simulink model "simsevenlevelmulti"  (R2023a)
settings: Solver=VariableStepAuto  StartTime=0.0  StopTime=10.0  RelTol=1e-3
libraries: spsIGBTDiodeLib x12, simulink x6, spsDCVoltageSourceLib x3, spsSeriesRLCBranchLib x1, spsVoltageMeasurementLib x1, spspowerguiLib x1
settings Model: Creator=banof  LastModifiedBy=banof

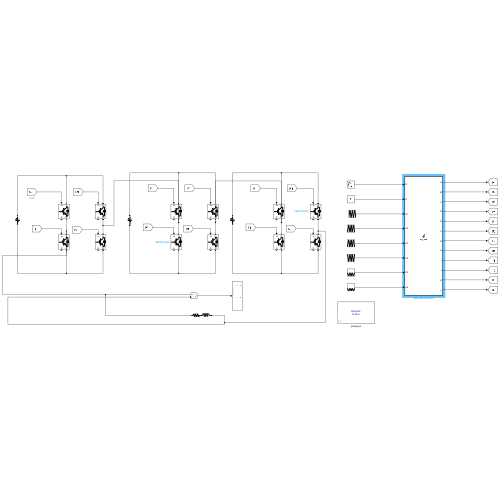
[thumbnail: Simulink's stored preview of the top-level diagram]
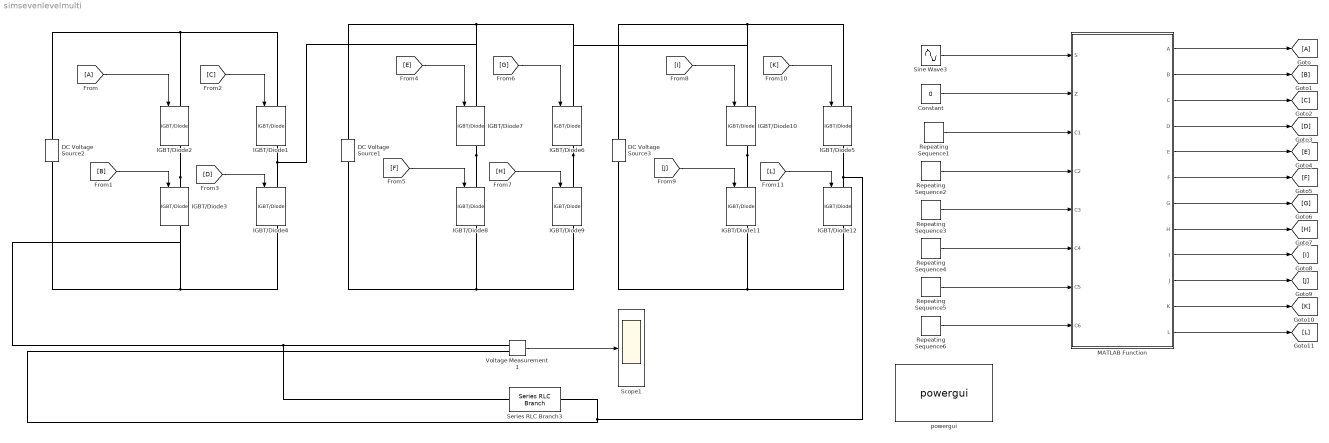
== system simsevenlevelmulti ==
  Constant : Constant  Value=0
  DC Voltage Source1 : spsDCVoltageSourceLib/DC Voltage Source  Amplitude=100  Measurements=None
  DC Voltage Source2 : spsDCVoltageSourceLib/DC Voltage Source  Amplitude=100  Measurements=None
  DC Voltage Source3 : spsDCVoltageSourceLib/DC Voltage Source  Amplitude=100  Measurements=None
  From : From
  Goto : Goto
  IGBT/Diode{1..12} (12 alike) : spsIGBTDiodeLib/IGBT//Diode  Ron=1e-3  Rs=1e5  Cs=inf  Measurements=on
  MATLAB Function : MATLAB Function  TreatAsAtomicUnit=on
  Repeating Sequence1 : simulink/Sources/Repeating Sequence  rep_seq_t=[0 0.5/1000 1/1000]  rep_seq_y=[0 0.3334 0]
  Repeating Sequence2 : simulink/Sources/Repeating Sequence  rep_seq_t=[0 0.5/1000 1/1000]  rep_seq_y=[0.3334 0.6667 0.3334]
  Repeating Sequence3 : simulink/Sources/Repeating Sequence  rep_seq_t=[0 0.5/1000 1/1000]  rep_seq_y=[0.6667 1.0000 0.6667]
  Repeating Sequence4 : simulink/Sources/Repeating Sequence  rep_seq_t=[0 0.5/1000 1/1000]  rep_seq_y=[0 -0.3334 0]
  Repeating Sequence5 : simulink/Sources/Repeating Sequence  rep_seq_t=[0 0.5/1000 1/1000]  rep_seq_y=[-0.3334 -0.6667 -0.3334]
  Repeating Sequence6 : simulink/Sources/Repeating Sequence  rep_seq_t=[0 0.5/1000 1/1000]  rep_seq_y=[-0.6667 -1 -0.6667]
  Scope1 : Scope
  Series RLC Branch3 : spsSeriesRLCBranchLib/Series RLC Branch  LConnTagsString=__new0  RConnTagsString=__new0  BranchType=RL  Resistance=100  Inductance=100e-3  SetiL0=off  InitialCurrent=0  Capacitance=1e-6  Setx0=off  InitialVoltage=0  Measurements=None
  Sine Wave3 : Sin  Frequency=2*pi*50
  Voltage Measurement1 : spsVoltageMeasurementLib/Voltage Measurement  PhasorSimulation=off  OutputType=Complex  PSBequivalent=0
  powergui : spspowerguiLib/powergui  Priority=1  SimulationMode=Discrete  SampleTime=1e-6  frequency=60  Iterations=50  frequencyindice=0  Pbase=100e6  ErrMax=1e-4  UnitsV=kV  UnitsW=MW  buscounter=0  FunctionMessages=off  echomessages=off  EnableUseOfTLC=off  CurrentSourceSwitches=off  DisableSnubberDevices=off  DisableRonSwitches=off  DisableVfSwitches=off  DisplayEquations=off  AutomaticDiscreteSolvers=off  SolverType=Tustin/Backward Euler (TBE)  Interpol=off  ExternalGateDelay=off  methode=off  Ts=100  x0status=blocks  SPID=on  SwTol=0  HookPort=off  NonlinearTolerance=1e-4  nMaxIteration=100  ContinueOnMaxIteration=off  RestoreLinks=warning  ResistiveCurrentMeasurement=off  Frange=[0:2:500]  Ylog=off  Xlog=on  ShowGrid=off  save=off  variable=ZData  structure=0  ZoomFFT=off  StartTime=0.0  cycles=1  DisplayStyle=1  fundamental=60  FreqAxis=off  MaxFrequency=1000  frequencyindicesteady=1  RmsSteady=1  display=off
  wires:
  MATLAB Function/2(B) -> [B]
  MATLAB Function/10(J) -> [J]
  MATLAB Function/8(H) -> [H]
  MATLAB Function/3(C) -> [C]
  MATLAB Function/1(A) -> Goto/1
  MATLAB Function/5(E) -> [E]
  Constant/1 -> MATLAB Function/2(Z)
  Repeating Sequence4/1 -> MATLAB Function/6(C4)
  Repeating Sequence1/1 -> MATLAB Function/3(C1)
  Repeating Sequence3/1 -> MATLAB Function/5(C3)
  MATLAB Function/12(L) -> [L]
  MATLAB Function/11(K) -> [K]
  Repeating Sequence2/1 -> MATLAB Function/4(C2)
  MATLAB Function/9(I) -> [I]
  Repeating Sequence6/1 -> MATLAB Function/8(C6)
  MATLAB Function/7(G) -> [G]
  MATLAB Function/4(D) -> [D]
  Sine Wave3/1 -> MATLAB Function/1(S)
  MATLAB Function/6(F) -> [F]
  Repeating Sequence5/1 -> MATLAB Function/7(C5)
  [C] -> IGBT/Diode1/1
  From/1 -> IGBT/Diode2/1
  [G] -> IGBT/Diode6/1
  [H] -> IGBT/Diode9/1
  [F] -> IGBT/Diode8/1
  [D] -> IGBT/Diode4/1
  [E] -> IGBT/Diode7/1
  [B] -> IGBT/Diode3/1
  Voltage Measurement1/1 -> Scope1/1
  [J] -> IGBT/Diode11/1
  [L] -> IGBT/Diode12/1
  [K] -> IGBT/Diode5/1
  [I] -> IGBT/Diode10/1
  connections:
  IGBT/Diode1/RConn1 -- IGBT/Diode8/LConn1 -- IGBT/Diode7/RConn1 -- IGBT/Diode4/LConn1
  IGBT/Diode6/LConn1 -- DC Voltage Source1/RConn1 -- IGBT/Diode7/LConn1
  IGBT/Diode4/RConn1 -- IGBT/Diode3/RConn1 -- DC Voltage Source2/LConn1
  Series RLC Branch3/LConn1 -- Voltage Measurement1/LConn1 -- IGBT/Diode2/RConn1 -- IGBT/Diode3/LConn1
  IGBT/Diode9/RConn1 -- IGBT/Diode8/RConn1 -- DC Voltage Source1/LConn1
  IGBT/Diode1/LConn1 -- DC Voltage Source2/RConn1 -- IGBT/Diode2/LConn1
  IGBT/Diode12/LConn1 -- IGBT/Diode5/RConn1 -- Voltage Measurement1/LConn2 -- Series RLC Branch3/RConn1
  IGBT/Diode12/RConn1 -- IGBT/Diode11/RConn1 -- DC Voltage Source3/LConn1
  IGBT/Diode9/LConn1 -- IGBT/Diode10/RConn1 -- IGBT/Diode11/LConn1 -- IGBT/Diode6/RConn1
  IGBT/Diode5/LConn1 -- DC Voltage Source3/RConn1 -- IGBT/Diode10/LConn1

== matlab function simsevenlevelmulti/MATLAB Function ==
  data: S input; A output; B output; C output; D output; E output; F output; G output; H output; I output; J output; K output; L output; Z input; C1 input; C2 input; C3 input; C4 input; C5 input; C6 input
function [A,B,C,D,E,F,G,H,I,J,K,L]= myfcn(S,Z,C1,C2,C3,C4,C5,C6)
    a=0;b=0;c=0;d=0;e=0;f=0;g=0;h=0;i=0;j=0;k=0;l=0;
if S>Z&&S>C1&&S<C2&&S<C3%1/3Vdc
    a=1;
    b=0;
    c=0;
    d=1;
    e=1;
    f=0;
    g=1;
    h=0;
    i=1;
    j=0;
    k=1;
    l=0;
elseif S>Z&&S>C1&&S>C2&&S<C3%2/3Vdc
    a=1;
    b=0;
    c=1;
    d=0;
    e=1;
    f=0;
    g=0;
    h=1;
    i=1;
    j=0;
    k=0;
    l=1;
elseif S>Z&&S>C1&&S>C2&&S>C3%VDC
    a=1;
    b=0;
    c=0;
    d=1;
    e=1;
    f=0;
    g=0;
    h=1;
    i=1;
    j=0;
    k=0;
    l=1;
  elseif S>Z&&S<C1&&S<C2&&S<C3%0Vdc
    a=1;
    b=0;
    c=1;
    d=0;
    e=1;
    f=0;
    g=1;
    h=0;    
    i=1;
    j=0;
    k=1;
    l=0;
elseif S<Z&&S>C4&&S>C5&&S>C6%0Vdc
    a=1;
    b=0;
    c=1;
    d=0;
    e=1;
    f=0;
    g=1;
    h=0;    
    i=1;
    j=0;
    k=1;
    l=0;
    elseif S<Z&&S<C4&&S>C5&&S>C6%-1/3Vdc
    a=0;
    b=1;
    c=1;
    d=0;
    e=1;
    f=0;
    g=1;
    h=0;    
    i=1;
    j=0;
    k=1;
    l=0;
    elseif S<Z&&S<C4&&S<C5&&S>C6%-2/3Vdc
    a=0;
    b=1;
    c=1;
    d=0;
    e=0;
    f=1;
    g=1;
    h=0;    
    i=1;
    j=0;
    k=1;
    l=0;
    elseif S<Z&&S<C4&&S<C5&&S<C6%-Vdc
    a=0;
    b=1;
    c=1;
    d=0;
    e=0;
    f=1;
    g=1;
    h=0;    
    i=0;
    j=1;
    k=1;
    l=0;
end
A=a;
B=b;
C=c;
D=d;
E=e;
F=f;
G=g;
H=h;
I=i;
J=j;
K=k;
L=l;
